simulink model "oppg1f"  (R2024a)
settings: Solver=ode1  StartTime=0.0  StopTime=15.0  FixedStep=0.1  RelTol=1e-3
settings Model: Creator=Lars André  LastModifiedBy=Lars André

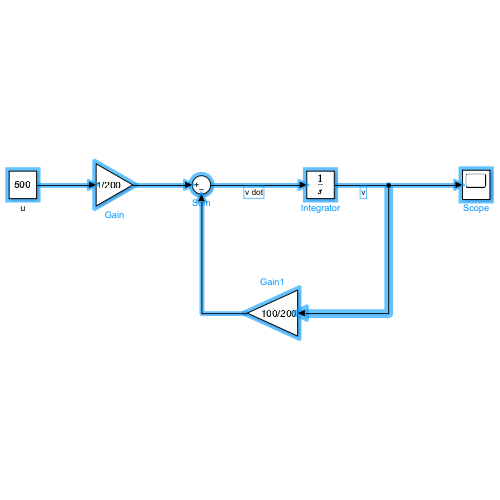
[thumbnail: Simulink's stored preview of the top-level diagram]
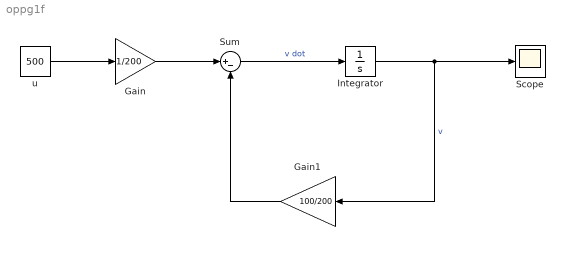
== system oppg1f ==
  Gain : Gain  Gain=1/200
  Gain1 : Gain  Gain=100/200
  Integrator : Integrator
  Scope : Scope
  Sum : Sum  Inputs=|+-
  u : Constant  Value=500
  wires:
  u/1 -> Gain/1
  Gain/1 -> Sum/1
  Sum/1 -> Integrator/1  "v dot"
  Integrator/1 -> Gain1/1, Scope/1  "v"
  Gain1/1 -> Sum/2
